simulink model "icecast_simevents"  (R2015a)
settings: Solver=FixedStepDiscrete  StartTime=0.0  StopTime=100000  RelTol=1e-3
libraries: simulink x2
settings Model: Creator=windor  LastModifiedBy=Ernesto Ardenghi

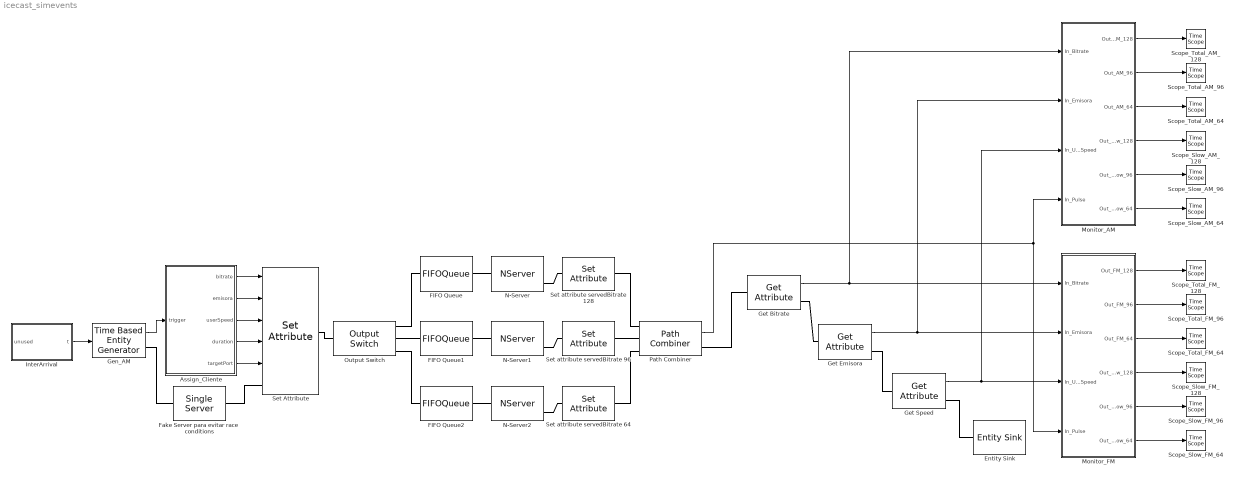
== system icecast_simevents ==
  Assign_Cliente : MATLAB Function  TreatAsAtomicUnit=on
  Entity Sink : EntitySink
  FIFO Queue : FIFOQueue
  FIFO Queue1 : FIFOQueue
  FIFO Queue2 : FIFOQueue
  Fake Server para evitar race conditions : SingleServer  ServiceTime=0
  Gen_AM : TimeBasedEntityGenerator  GenerateEntitiesUpon=Intergeneration time from port t  StatNumberDeparted=on
  Get Bitrate : GetAttribute  AttributeName=servedBitrate  EvaluatedDefaultAttributeValue={ []}
      settings: OutputPortMap=o1
  Get Emisora : GetAttribute  AttributeName=emisora  EvaluatedDefaultAttributeValue={ []}
      settings: OutputPortMap=o1
  Get Speed : GetAttribute  AttributeName=userSpeed  EvaluatedDefaultAttributeValue={ []}
      settings: OutputPortMap=o1
  InterArrival : MATLAB Function  TreatAsAtomicUnit=on
  Monitor_AM : Subsystem
  Monitor_FM : Subsystem
  N-Server : NServer  ServiceTimeFrom=Attribute  AttributeName=duration  StatNumberDeparted=on
  N-Server1 : NServer  ServiceTimeFrom=Attribute  AttributeName=duration  StatNumberDeparted=on
  N-Server2 : NServer  ServiceTimeFrom=Attribute  AttributeName=duration  StatNumberDeparted=on
  Output Switch : OutputSwitch  SwitchingCriterion=From attribute  AttributeName=targetPort
  Path Combiner : PathCombiner  StatNumberDeparted=on
  Scope_Slow_AM_128 : TimeScope
  Scope_Slow_AM_64 : TimeScope
  Scope_Slow_AM_96 : TimeScope
  Scope_Slow_FM_128 : TimeScope
  Scope_Slow_FM_64 : TimeScope
  Scope_Slow_FM_96 : TimeScope
  "Scope_Total_AM_128 " : TimeScope
  Scope_Total_AM_64 : TimeScope
  Scope_Total_AM_96 : TimeScope
  Scope_Total_FM_128 : TimeScope
  Scope_Total_FM_64 : TimeScope
  Scope_Total_FM_96 : TimeScope
  Set Attribute : SetAttribute  AttributeName=bitrate|emisora|userSpeed|duration|targetPort  AttributeFrom=Signal port|Signal port|Signal port|Signal port|Signal port  AttributeValue=1|1|1|1|1  AttributeTreatAsVector=0|1|1|0|1  EvaluatedAttributeValue={ [];[];[];[];[]}
      settings: InputPortMap=u0,u1,u2,u3,u4
  Set attribute servedBitrate 128 : SetAttribute  AttributeName=servedBitrate  AttributeValue=128  AttributeTreatAsVector=0  EvaluatedAttributeValue={ 128}
  Set attribute servedBitrate 64 : SetAttribute  AttributeName=servedBitrate  AttributeValue=64  EvaluatedAttributeValue={ 64}
  Set attribute servedBitrate 96 : SetAttribute  AttributeName=servedBitrate  AttributeValue=96  EvaluatedAttributeValue={ 96}
  wires:
  InterArrival/1(t) -> Gen_AM/1
  Gen_AM/1 -> Assign_Cliente/1(trigger)
  Get Bitrate/1 -> Monitor_FM/1(In_Bitrate), Monitor_AM/1(In_Bitrate)
  Get Emisora/1 -> Monitor_FM/2(In_Emisora), Monitor_AM/2(In_Emisora)
  Get Speed/1 -> Monitor_FM/3(In_UserSpeed), Monitor_AM/3(In_UserSpeed)
  Path Combiner/1 -> Monitor_FM/4(In_Pulse), Monitor_AM/4(In_Pulse)
  Monitor_AM/1(Out_AM_128) -> "Scope_Total_AM_128 "/1
  Monitor_AM/4(Out_AM_Slow_128) -> Scope_Slow_AM_128/1
  Monitor_AM/2(Out_AM_96) -> Scope_Total_AM_96/1
  Monitor_AM/3(Out_AM_64) -> Scope_Total_AM_64/1
  Monitor_AM/5(Out_AM_Slow_96) -> Scope_Slow_AM_96/1
  Monitor_AM/6(Out_AM_Slow_64) -> Scope_Slow_AM_64/1
  Monitor_FM/1(Out_FM_128) -> Scope_Total_FM_128/1
  Monitor_FM/2(Out_FM_96) -> Scope_Total_FM_96/1
  Monitor_FM/3(Out_FM_64) -> Scope_Total_FM_64/1
  Monitor_FM/4(Out_FM_Slow_128) -> Scope_Slow_FM_128/1
  Monitor_FM/5(Out_FM_Slow_96) -> Scope_Slow_FM_96/1
  Monitor_FM/6(Out_FM_Slow_64) -> Scope_Slow_FM_64/1
  Assign_Cliente/1(bitrate) -> Set Attribute/1
  Assign_Cliente/2(emisora) -> Set Attribute/2
  Assign_Cliente/3(userSpeed) -> Set Attribute/3
  Assign_Cliente/4(duration) -> Set Attribute/4
  Assign_Cliente/5(targetPort) -> Set Attribute/5
  connections:
  Get Bitrate/RConn1 -- Get Emisora/LConn1
  Get Emisora/RConn1 -- Get Speed/LConn1
  N-Server/LConn1 -- FIFO Queue/RConn1
  Gen_AM/RConn1 -- Fake Server para evitar race conditions/LConn1
  Fake Server para evitar race conditions/RConn1 -- Set Attribute/LConn1
  Output Switch/LConn1 -- Set Attribute/RConn1
  Output Switch/RConn1 -- FIFO Queue/LConn1
  Output Switch/RConn2 -- FIFO Queue1/LConn1
  Output Switch/RConn3 -- FIFO Queue2/LConn1
  N-Server1/LConn1 -- FIFO Queue1/RConn1
  N-Server2/LConn1 -- FIFO Queue2/RConn1
  N-Server1/RConn1 -- Set attribute servedBitrate 96/LConn1
  N-Server2/RConn1 -- Set attribute servedBitrate 64/LConn1
  N-Server/RConn1 -- Set attribute servedBitrate 128/LConn1
  Set attribute servedBitrate 96/RConn1 -- Path Combiner/LConn2
  Set attribute servedBitrate 128/RConn1 -- Path Combiner/LConn1
  Set attribute servedBitrate 64/RConn1 -- Path Combiner/LConn3
  Get Bitrate/LConn1 -- Path Combiner/RConn1
  Get Speed/RConn1 -- Entity Sink/LConn1

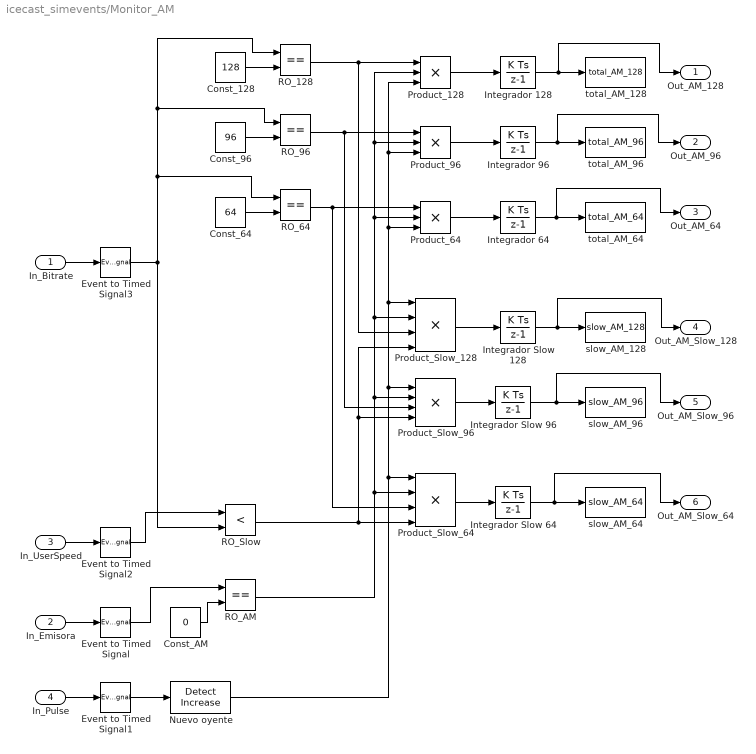
== system icecast_simevents/Monitor_AM ==
  In_Bitrate : Inport
  In_Emisora : Inport  Port=2
  In_UserSpeed : Inport  Port=3
  In_Pulse : Inport  Port=4
  Const_128 : Constant  Value=128  VectorParams1D=off
  Const_64 : Constant  Value=64  VectorParams1D=off
  Const_96 : Constant  Value=96  VectorParams1D=off
  Const_AM : Constant  Value=0
  Event to Timed Signal{,1..3} (4 alike) : EventToTimedSignal
  Integrador Slow 64 : DiscreteIntegrator  InitialConditionSetting=State (most efficient)
  Integrador Slow 96 : DiscreteIntegrator  InitialConditionSetting=State (most efficient)
  Integrador Slow 128 : DiscreteIntegrator  InitialConditionSetting=State (most efficient)
  Integrador 128 : DiscreteIntegrator  InitialConditionSetting=State (most efficient)
  Integrador 64 : DiscreteIntegrator  InitialConditionSetting=State (most efficient)
  Integrador 96 : DiscreteIntegrator  InitialConditionSetting=State (most efficient)
  Nuevo oyente : simulink/Logic and Bit Operations/Detect Increase  vinit=0.0  InputProcessing=Inherited  OutDataTypeStr=boolean
  Product_128 : Product  Inputs=3
  Product_64 : Product  Inputs=3
  Product_96 : Product  Inputs=3
  Product_Slow_128 : Product  Inputs=4
  Product_Slow_64 : Product  Inputs=4
  Product_Slow_96 : Product  Inputs=4
  RO_128 : RelationalOperator  Operator===  OutDataTypeStr=boolean
  RO_64 : RelationalOperator  Operator===  OutDataTypeStr=boolean
  RO_96 : RelationalOperator  Operator===  OutDataTypeStr=boolean
  RO_AM : RelationalOperator  Operator===  OutDataTypeStr=boolean
  "RO_Slow " : RelationalOperator  Operator=<  OutDataTypeStr=boolean
  slow_AM_128 : ToWorkspace  VariableName=slow_AM_128  SaveFormat=Timeseries  SampleTime=-1
  slow_AM_64 : ToWorkspace  VariableName=slow_AM_64  SaveFormat=Timeseries  SampleTime=-1
  slow_AM_96 : ToWorkspace  VariableName=slow_AM_96  SaveFormat=Timeseries  SampleTime=-1
  total_AM_128 : ToWorkspace  VariableName=total_AM_128  SaveFormat=Timeseries  SampleTime=-1
  total_AM_64 : ToWorkspace  VariableName=total_AM_64  SaveFormat=Timeseries  SampleTime=-1
  total_AM_96 : ToWorkspace  VariableName=total_AM_96  SaveFormat=Timeseries  SampleTime=-1
  Out_AM_128 : Outport
  Out_AM_96 : Outport  Port=2
  Out_AM_64 : Outport  Port=3
  Out_AM_Slow_128 : Outport  Port=4
  Out_AM_Slow_96 : Outport  Port=5
  Out_AM_Slow_64 : Outport  Port=6
  wires:
  Const_AM/1 -> RO_AM/2
  In_Bitrate/1 -> Event to Timed Signal3/1
  In_Emisora/1 -> Event to Timed Signal/1
  In_UserSpeed/1 -> Event to Timed Signal2/1
  "RO_Slow "/1 -> Product_Slow_64/4, Product_Slow_96/4, Product_Slow_128/4
  In_Pulse/1 -> Event to Timed Signal1/1
  Event to Timed Signal1/1 -> Nuevo oyente/1
  Nuevo oyente/1 -> Product_96/3, Product_128/3, Product_64/3, Product_Slow_128/1, Product_Slow_96/1, Product_Slow_64/1
  Event to Timed Signal3/1 -> RO_128/1, RO_96/1, RO_64/1, "RO_Slow "/2
  Event to Timed Signal/1 -> RO_AM/1
  Event to Timed Signal2/1 -> "RO_Slow "/1
  RO_AM/1 -> Product_Slow_64/2, Product_Slow_96/2, Product_96/2, Product_128/2, Product_64/2, Product_Slow_128/2
  Const_128/1 -> RO_128/2
  Const_96/1 -> RO_96/2
  Const_64/1 -> RO_64/2
  RO_128/1 -> Product_Slow_128/3, Product_128/1
  RO_96/1 -> Product_Slow_96/3, Product_96/1
  RO_64/1 -> Product_Slow_64/3, Product_64/1
  Product_128/1 -> Integrador 128/1
  Product_96/1 -> Integrador 96/1
  Product_64/1 -> Integrador 64/1
  Integrador 128/1 -> Out_AM_128/1, total_AM_128/1
  Integrador 96/1 -> Out_AM_96/1, total_AM_96/1
  Integrador 64/1 -> Out_AM_64/1, total_AM_64/1
  Product_Slow_128/1 -> Integrador Slow 128/1
  Integrador Slow 128/1 -> Out_AM_Slow_128/1, slow_AM_128/1
  Product_Slow_96/1 -> Integrador Slow 96/1
  Integrador Slow 96/1 -> Out_AM_Slow_96/1, slow_AM_96/1
  Product_Slow_64/1 -> Integrador Slow 64/1
  Integrador Slow 64/1 -> Out_AM_Slow_64/1, slow_AM_64/1

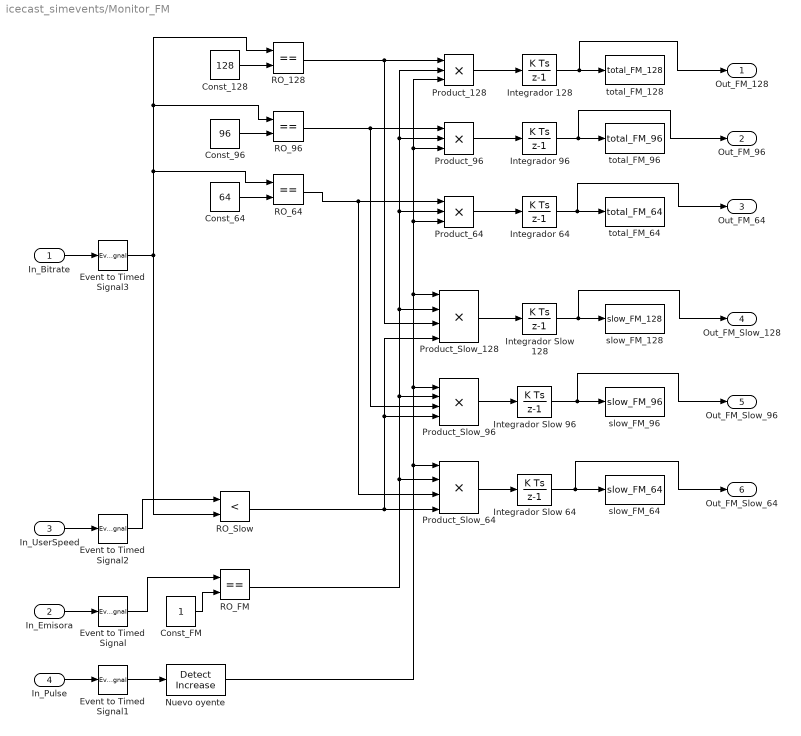
== system icecast_simevents/Monitor_FM ==
  In_Bitrate : Inport
  In_Emisora : Inport  Port=2
  In_UserSpeed : Inport  Port=3
  In_Pulse : Inport  Port=4
  Const_128 : Constant  Value=128  VectorParams1D=off
  Const_64 : Constant  Value=64  VectorParams1D=off
  Const_96 : Constant  Value=96  VectorParams1D=off
  Const_FM : Constant
  Event to Timed Signal{,1..3} (4 alike) : EventToTimedSignal
  Integrador Slow 64 : DiscreteIntegrator  InitialConditionSetting=State (most efficient)
  Integrador Slow 96 : DiscreteIntegrator  InitialConditionSetting=State (most efficient)
  Integrador Slow 128 : DiscreteIntegrator  InitialConditionSetting=State (most efficient)
  Integrador 128 : DiscreteIntegrator  InitialConditionSetting=State (most efficient)
  Integrador 64 : DiscreteIntegrator  InitialConditionSetting=State (most efficient)
  Integrador 96 : DiscreteIntegrator  InitialConditionSetting=State (most efficient)
  Nuevo oyente : simulink/Logic and Bit Operations/Detect Increase  vinit=0.0  InputProcessing=Inherited  OutDataTypeStr=boolean
  Product_128 : Product  Inputs=3
  Product_64 : Product  Inputs=3
  Product_96 : Product  Inputs=3
  Product_Slow_128 : Product  Inputs=4
  Product_Slow_64 : Product  Inputs=4
  Product_Slow_96 : Product  Inputs=4
  RO_128 : RelationalOperator  Operator===  OutDataTypeStr=boolean
  RO_64 : RelationalOperator  Operator===  OutDataTypeStr=boolean
  RO_96 : RelationalOperator  Operator===  OutDataTypeStr=boolean
  RO_FM : RelationalOperator  Operator===  OutDataTypeStr=boolean
  "RO_Slow " : RelationalOperator  Operator=<  OutDataTypeStr=boolean
  slow_FM_128 : ToWorkspace  VariableName=slow_FM_128  SaveFormat=Timeseries  SampleTime=-1
  slow_FM_64 : ToWorkspace  VariableName=slow_FM_64  SaveFormat=Timeseries  SampleTime=-1
  slow_FM_96 : ToWorkspace  VariableName=slow_FM_96  SaveFormat=Timeseries  SampleTime=-1
  "total_FM_128 " : ToWorkspace  VariableName=total_FM_128  SaveFormat=Timeseries  SampleTime=-1
  total_FM_64 : ToWorkspace  VariableName=total_FM_64  SaveFormat=Timeseries  SampleTime=-1
  total_FM_96 : ToWorkspace  VariableName=total_FM_96  SaveFormat=Timeseries  SampleTime=-1
  Out_FM_128 : Outport
  Out_FM_96 : Outport  Port=2
  Out_FM_64 : Outport  Port=3
  Out_FM_Slow_128 : Outport  Port=4
  Out_FM_Slow_96 : Outport  Port=5
  Out_FM_Slow_64 : Outport  Port=6
  wires:
  Const_FM/1 -> RO_FM/2
  In_Bitrate/1 -> Event to Timed Signal3/1
  In_Emisora/1 -> Event to Timed Signal/1
  In_UserSpeed/1 -> Event to Timed Signal2/1
  "RO_Slow "/1 -> Product_Slow_64/4, Product_Slow_128/4, Product_Slow_96/4
  In_Pulse/1 -> Event to Timed Signal1/1
  Event to Timed Signal1/1 -> Nuevo oyente/1
  Nuevo oyente/1 -> Product_96/3, Product_128/3, Product_64/3, Product_Slow_128/1, Product_Slow_96/1, Product_Slow_64/1
  Event to Timed Signal3/1 -> RO_128/1, RO_96/1, RO_64/1, "RO_Slow "/2
  Event to Timed Signal/1 -> RO_FM/1
  Event to Timed Signal2/1 -> "RO_Slow "/1
  RO_FM/1 -> Product_Slow_64/2, Product_96/2, Product_128/2, Product_64/2, Product_Slow_128/2, Product_Slow_96/2
  Const_128/1 -> RO_128/2
  Const_96/1 -> RO_96/2
  Const_64/1 -> RO_64/2
  RO_128/1 -> Product_Slow_128/3, Product_128/1
  RO_96/1 -> Product_Slow_96/3, Product_96/1
  RO_64/1 -> Product_Slow_64/3, Product_64/1
  Product_128/1 -> Integrador 128/1
  Product_96/1 -> Integrador 96/1
  Product_64/1 -> Integrador 64/1
  Integrador 128/1 -> Out_FM_128/1, "total_FM_128 "/1
  Integrador 96/1 -> Out_FM_96/1, total_FM_96/1
  Integrador 64/1 -> Out_FM_64/1, total_FM_64/1
  Product_Slow_128/1 -> Integrador Slow 128/1
  Integrador Slow 128/1 -> Out_FM_Slow_128/1, slow_FM_128/1
  Product_Slow_96/1 -> Integrador Slow 96/1
  Integrador Slow 96/1 -> Out_FM_Slow_96/1, slow_FM_96/1
  Product_Slow_64/1 -> Integrador Slow 64/1
  Integrador Slow 64/1 -> Out_FM_Slow_64/1, slow_FM_64/1

== matlab function icecast_simevents/InterArrival ==
  data: unused input; t output
function t = InterArrival_General(~)
% Generado por bootstrap_inicial.m - 03-Feb-2026 14:30:25
persistent init mu_log sigma_log;
if isempty(init)
    mu_log = 3.489800;
    sigma_log = 0.802600;
    init = 1;
end
t = lognrnd(mu_log, sigma_log);
if t <= 0 || t > 3600
    t = 10;
end
end

== matlab function icecast_simevents/Assign_Cliente ==
  data: bitrate output double; emisora output double; trigger input double; userSpeed output double; duration output double; targetPort output
function [bitrate, emisora, userSpeed, duration, targetPort] = Assign_Cliente(trigger)
%% Generado por iniciar_presimulacion.m - MODO RUTEO INTELIGENTE
persistent init prob_AM prob_slow_AM prob_slow_FM;
if isempty(init)
    prob_AM = 0.755356;
    prob_slow_AM = 0.007112;
    prob_slow_FM = 0.002006;
    init = 1;
end

%% 1. Asignar Emisora (Igual que antes)
r = rand();
if r < prob_AM
    emisora = 0; %% AM
else
    emisora = 1; %% FM
end

%% 2. Asignar userSpeed (MOVIDO AL PRINCIPIO)
% Primero medimos "cuánto internet tiene el usuario"
if emisora == 0
    if rand() < prob_slow_AM
        userSpeed = round(normrnd(80, 20));
        if userSpeed <= 0, userSpeed = 50; end
    else
        userSpeed = round(normrnd(160, 30));
    end
else
    if rand() < prob_slow_FM
        userSpeed = round(normrnd(80, 20));
        if userSpeed <= 0, userSpeed = 50; end
    else
        userSpeed = round(normrnd(160, 30));
    end
end

%% 3. Asignar Bitrate y TargetPort (LÓGICA INTELIGENTE)
% Aquí ocurre la magia: Le damos la mejor calidad posible SIN que se corte.

% Margen de seguridad: El usuario debe tener al menos la velocidad del stream.
if userSpeed >= 128
    % Si tiene buen internet, le damos HD
    bitrate = 128;
    targetPort = 1;
elseif userSpeed >= 96
    % Si no llega a HD pero es decente, le damos Media
    bitrate = 96;
    targetPort = 2;
else
    % Si su internet es malo, le damos Baja para evitar cortes
    bitrate = 64;
    targetPort = 3;
end

%% 4. Asignar duration (Igual que antes)
if emisora == 0
    duration = round(normrnd(300, 60));
else
    duration = round(normrnd(240, 40));
end
if duration <= 0
    duration = 60;
end
end
